simulink model "Simulink_Model_1"  (R2025b)
settings: Solver=ode23  StartTime=0.0  StopTime=50  FixedStep=0.01  MaxStep=1.0  RelTol=1e-3
libraries: simulink_extras x1
settings Model: Creator=dburl  LastModifiedBy=dburl

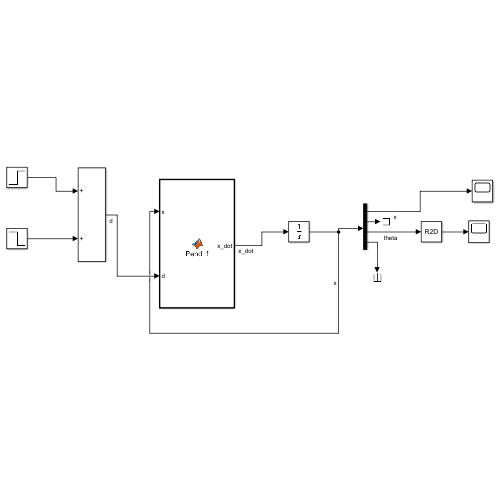
[thumbnail: Simulink's stored preview of the top-level diagram]
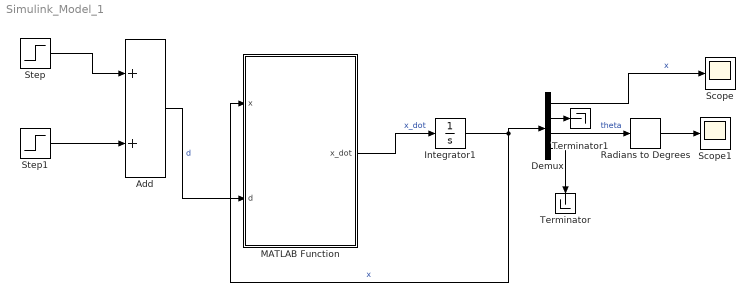
== system Simulink_Model_1 ==
  Add : Sum
  Demux : Demux
  Integrator1 : Integrator  InitialCondition=[0;0;0;0]
  MATLAB Function : MATLAB Function  TreatAsAtomicUnit=on
  Radians to Degrees : simulink_extras/Transformations/Radians to Degrees
  Scope : Scope
      settings: ActiveDisplayYMinimum=-1  ActiveDisplayYMaximum=1
  Scope1 : Scope
      settings: ActiveDisplayYMinimum=-1  ActiveDisplayYMaximum=1
  Step : Step  SampleTime=0
  Step1 : Step  Time=3  After=-1  SampleTime=0
  Terminator : Terminator
  Terminator1 : Terminator
  wires:
  Step/1 -> Add/1
  Step1/1 -> Add/2
  Integrator1/1 -> Demux/1, MATLAB Function/1(x)  "x"
  Add/1 -> MATLAB Function/2(d)  "d"
  MATLAB Function/1(x_dot) -> Integrator1/1  "x_dot"
  Demux/1 -> Scope/1  "x"
  Demux/3 -> Radians to Degrees/1  "theta"
  Demux/4 -> Terminator/1
  Demux/2 -> Terminator1/1
  Radians to Degrees/1 -> Scope1/1

== matlab function Simulink_Model_1/MATLAB Function ==
  data: x_dot output; x input; d input; Pend parameter
function x_dot  = Pend_f(x,d, Pend)
M = Pend.M;
m = Pend.m;
l = Pend.l;
g = Pend.g;
c = Pend.c;
b = Pend.b;
d0 = Pend.d0;
x1 = x(1);
x2 = x(2);
x3 = x(3);
x4 = x(4);

%abbiamo assunto i(t) = 0
xdot1 = x2;
xdot2 = (1/2*m*l*cos(x3)*((m*g*l/2)*sin(x3)-b*x4+d0*d*l^2/2*cos(x3))+1/3*m*l^2 ...
    *(-1/2*m*l*(x4)^2*sin(x3)-c*x2-d0*l*d))/(1/3*m*(M+m)*l^2-1/4*m^2*l^2*cos(x3)^2);
xdot3 = x4;
xdot4 = ((M+m)*(m*g*l/2*sin(x3)-b*x4+d0*d*l^2/2*cos(x3))+1/2*m*l*cos(x3)*...
    (-1/2*m*l*(x4)^2*sin(x3)-c*x2-d0*l*d))/(1/3*m*(M+m)*l^2-1/4*m^2*l^2*cos(x3)^2);
x_dot = [xdot1;xdot2;xdot3;xdot4];

end
